simulink model "finModelTest"  (R2025b)
settings: Solver=VariableStepAuto  StartTime=0.0  StopTime=10.0  RelTol=1e-3
settings Model: PauseTimes=0  Creator=maxhu  LastModifiedBy=maxhu

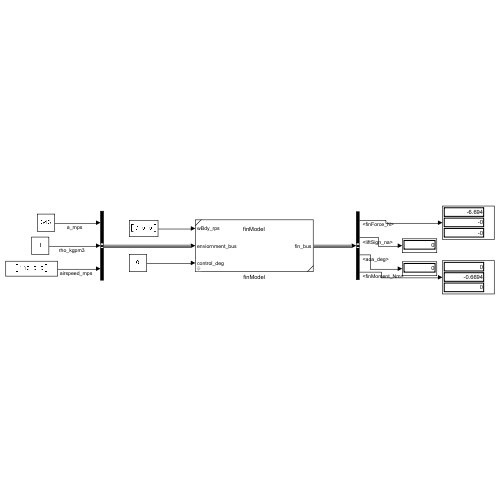
[thumbnail: Simulink's stored preview of the top-level diagram]
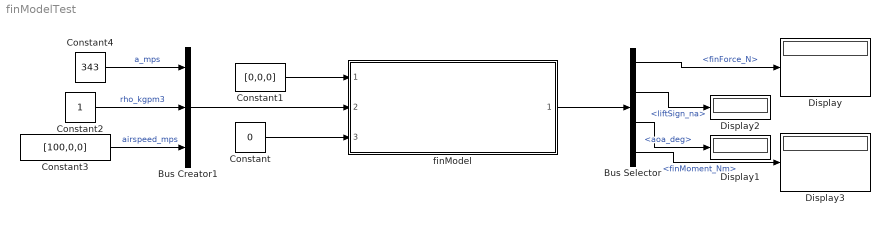
== system finModelTest ==
  Bus Creator1 : BusCreator  Inputs=3
  Bus Selector : BusSelector  OutputSignals=finForce_N,liftSign_na,aoa_deg,finMoment_Nm
  Constant : Constant  Value=0
  Constant1 : Constant  Value=[0,0,0]
  Constant2 : Constant
  Constant3 : Constant  Value=[100,0,0]
  Constant4 : Constant  Value=343
  Display{,1..3} (4 alike) : Display
  finModel : Subsystem  ReferencedSubsystem=finModel  finAngles_rad=[pi/2, 0, 0]  finMomentArm_m=[-1,0,0.1]
      settings: PermitHierarchicalResolution=None
  wires:
  Constant1/1 -> finModel/1
  Bus Creator1/1 -> finModel/2
  Bus Selector/1 -> Display/1  "<finForce_N>"
  Constant4/1 -> Bus Creator1/1  "a_mps"
  finModel/1 -> Bus Selector/1
  Constant2/1 -> Bus Creator1/2  "rho_kgpm3"
  Constant/1 -> finModel/3
  Constant3/1 -> Bus Creator1/3  "airspeed_mps"
  Bus Selector/3 -> Display1/1  "<aoa_deg>"
  Bus Selector/2 -> Display2/1  "<liftSign_na>"
  Bus Selector/4 -> Display3/1  "<finMoment_Nm>"
